simulink model "helicopter_auto_mode"  (Simulink 7.5)
settings: Solver=ode1  StartTime=0.0  StopTime=inf  FixedStep=0.1  RelTol=1e-3
PreLoadFcn:
  | load(fullfile(fileparts(which(bdroot)), 'object_types.mat'));
InitFcn:
  | load(fullfile(fileparts(which(bdroot)), 'object_types.mat'));
undefined symbols (not defined in the file or in its folder): HIL
libraries: quarc_library x4, simulink x1
settings Model: Creator=ovidiua  LastModifiedBy=ovidiua  SimulationMode=external  ExtModeTrigDuration=5000
settings SolverCC: PositivePriorityOrder=on
settings RTWCC: SystemTargetFile=quarc_windows.tlc  TemplateMakefile=quarc_default_tmf  Description=QUARC Win32 Target  ProcessScript=quarc_windows_make_rtw_hook
settings STFCustomTargetCC: TargetPreCompLibLocation=C:\PROGRA~2\QUARC\lib\2010a\windows\release  GeneratePreprocessorConditionals=Disable all  SystemTargetFile=quarc_windows.tlc
settings GRTTargetCC: TargetPreCompLibLocation=C:\PROGRA~2\QUARC\lib\2010a\windows\release  ParMdlRefBuildCompliant=off  CompOptLevelCompliant=off  MatFileLogging=off  ExtMode=on  ExtModeMexFile=quarc_comm

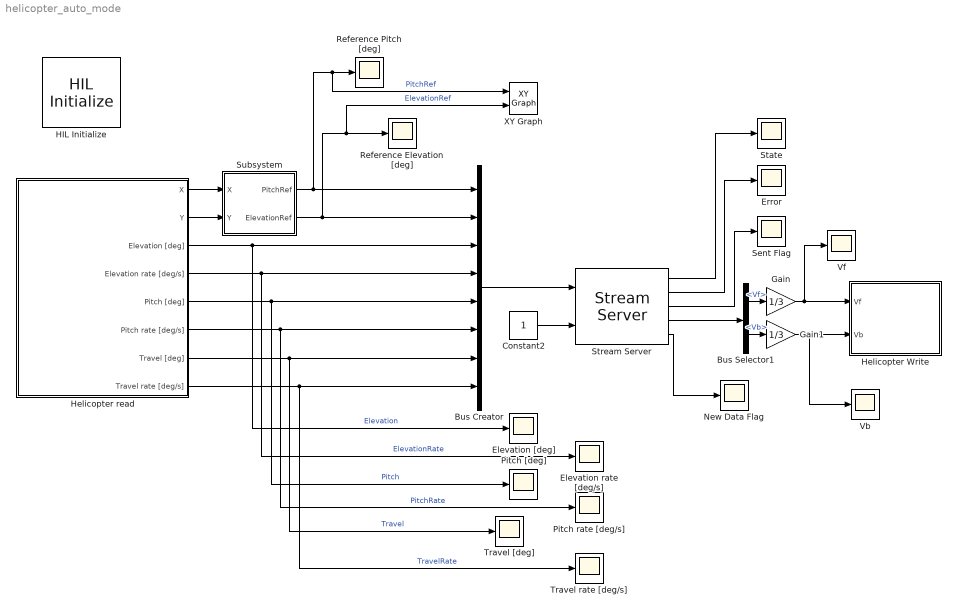
== system helicopter_auto_mode ==
  Bus Creator : BusCreator  Inputs='PitchRef','ElevationRef','Elevation','ElevationRate','Pitch','PitchRate','Travel','TravelRate'  UseBusObject=on
      settings: BusObject=BusObjectStates
  Bus Selector1 : BusSelector  OutputSignals=Vf,Vb
  Constant2 : Constant  OutDataType=sfix(16)  OutScaling=2^0
  Elevation [deg] : Scope
      settings: TimeRange=60  YMin=-30  YMax=30  SaveName=ScopeData2
  Elevation rate [deg/s] : Scope
      settings: TimeRange=60  YMin=-100  YMax=100  SaveName=ScopeData5
  Error : Scope
      settings: YMin=-1  YMax=1  SaveName=ScopeData8
  Gain : Gain  Gain=1/3  ParameterDataType=fixdt(1, 16)  ParameterScaling=2^0  OutDataType=fixdt(1, 16)  OutScaling=2^0
  Gain1 : Gain  Gain=1/3  ParameterDataType=fixdt(1, 16)  ParameterScaling=2^0  OutDataType=fixdt(1, 16)  OutScaling=2^0
  HIL Initialize : quarc_library/Data Acquisition/Generic/Configuration/HIL Initialize  object_name=HIL-1  board_type=q4  board_number=0  exclusive=off  active=off  hardware_clocks=[0:1]  clock_modes=[0 0]  set_clock_params_at_start=on  set_clock_params_at_switch_in=off  analog_input_channels=[0:3]  analog_input_maximums=10  analog_input_minimums=-10  set_analog_input_params_at_start=off  set_analog_input_params_at_switch_in=off  analog_output_channels=[0:3]  analog_output_maximums=[10]  analog_output_minimums=[-10]  initial_analog_outputs=[0]  final_analog_outputs=[0]  watchdog_analog_outputs=0  set_analog_output_params_at_start=on  set_analog_output_params_at_switch_in=off  set_analog_outputs_at_start=on  set_analog_outputs_at_switch_in=off  set_analog_outputs_at_terminate=on  set_analog_outputs_at_switch_out=off  set_analog_outputs_on_watchdog=off  digital_input_channels=[]  digital_output_channels=[]  digital_output_configuration=[]  initial_digital_outputs=[1]  final_digital_outputs=[1]  watchdog_digital_outputs=[2]  set_digital_output_params_at_start=off  set_digital_output_params_at_switch_in=off  set_digital_outputs_at_start=on  set_digital_outputs_at_switch_in=off  set_digital_outputs_at_terminate=on  set_digital_outputs_at_switch_out=off  set_digital_outputs_on_watchdog=off  encoder_channels=[0:3]  quadrature=[4]  encoder_filter_frequency=(1/60e-9)/1  initial_encoder_counts=[0]  set_encoder_params_at_start=on  set_encoder_params_at_switch_in=off  set_encoder_counts_at_start=on  set_encoder_counts_at_switch_in=off  pwm_channels=[]  pwm_modes=[0]  pwm_frequency=(1/60e-9)/1024  pwm_configuration=[]  pwm_alignment=[]  pwm_polarity=[]  pwm_leading_deadband=[]  pwm_trailing_deadband=[]  initial_pwm_outputs=[0]  final_pwm_outputs=[0]  watchdog_pwm_outputs=[]  set_pwm_params_at_start=on  set_pwm_params_at_switch_in=off  set_pwm_outputs_at_start=on  set_pwm_outputs_at_switch_in=off  set_pwm_outputs_at_terminate=on  set_pwm_outputs_at_switch_out=off  set_pwm_outputs_on_watchdog=off  other_output_channels=[]  initial_other_outputs=[]  final_other_outputs=[]  watchdog_other_outputs=[]  set_other_outputs_at_start=off  set_other_outputs_at_switch_in=off  set_other_outputs_at_terminate=off  set_other_outputs_at_switch_out=off  set_other_outputs_on_watchdog=off
  Helicopter Write : Subsystem
  Helicopter read : Subsystem
  New Data Flag : Scope
      settings: YMin=-1  YMax=1  SaveName=ScopeData9
  Pitch [deg] : Scope
      settings: TimeRange=60  YMin=-60  YMax=60  SaveName=ScopeData3
  Pitch rate [deg/s] : Scope
      settings: TimeRange=60  YMin=-100  YMax=100  SaveName=ScopeData6
  Reference Elevation [deg] : Scope
      settings: YMin=-3.75  YMax=-0.5
  Reference Pitch [deg] : Scope
      settings: YMin=-27.5  YMax=0
  Sent Flag : Scope
      settings: SaveName=ScopeData12
  State : Scope
      settings: YMin=-1  YMax=1  SaveName=ScopeData13
  Stream Server : quarc_library/Communications/Basic/Stream Server  uri_source=Specify via dialog (do not evaluate)  uri=shmem://foobar:1  apply_uri_to_all_configs=on  send_buffer_size=1460  receive_buffer_size=1460  byte_order=little endian (Intel - LSB first)  optimization=Minimum latency  implementation=Use blocking I/O in a separate thread  send_options=Send most recent data  receive_options=Receive most recent data  send_fifo_size=1000  receive_fifo_size=1000  send_priority=0  receive_priority=0  default_value=default_inputs  sample_time=qc_get_step_size  active=on  data_type=Specify via dialog  type_expr=BusObjectIn
      settings: AttributesFormatString="\"shmem://foobar:1\""
  Subsystem : Subsystem
  Travel [deg] : Scope
      settings: TimeRange=60  YMin=-360  YMax=360  SaveName=ScopeData4
  Travel rate [deg/s] : Scope
      settings: TimeRange=60  YMin=-100  YMax=100  SaveName=ScopeData7
  Vb : Scope
      settings: YMin=-22.5  YMax=20  SaveName=ScopeData11
  Vf : Scope
      settings: YMin=-80  YMax=70  SaveName=ScopeData10
  XY Graph : simulink/Sinks/XY Graph  SystemSampleTime=-1  xmin=-60  xmax=60  ymin=-30  ymax=30  st=-1
  wires:
  Subsystem/1(PitchRef) -> Bus Creator/1, Reference Pitch [deg]/1, XY Graph/1  "PitchRef"
  Subsystem/2(ElevationRef) -> Bus Creator/2, Reference Elevation [deg]/1, XY Graph/2  "ElevationRef"
  Helicopter read/3(Elevation [deg]) -> Elevation [deg]/1, Bus Creator/3  "Elevation"
  Helicopter read/4(Elevation rate [deg/s]) -> Elevation rate [deg/s]/1, Bus Creator/4  "ElevationRate"
  Helicopter read/5(Pitch [deg]) -> Pitch [deg]/1, Bus Creator/5  "Pitch"
  Helicopter read/6(Pitch rate [deg/s]) -> Pitch rate [deg/s]/1, Bus Creator/6  "PitchRate"
  Helicopter read/7(Travel [deg]) -> Travel [deg]/1, Bus Creator/7  "Travel"
  Helicopter read/8(Travel rate [deg/s]) -> Travel rate [deg/s]/1, Bus Creator/8  "TravelRate"
  Stream Server/1 -> State/1
  Stream Server/2 -> Error/1
  Constant2/1 -> Stream Server/2
  Bus Creator/1 -> Stream Server/1
  Stream Server/3 -> Sent Flag/1
  Stream Server/5 -> New Data Flag/1
  Stream Server/4 -> Bus Selector1/1
  Bus Selector1/1 -> Gain/1  "<Vf>"
  Bus Selector1/2 -> Gain1/1  "<Vb>"
  Helicopter read/1(X) -> Subsystem/1(X)
  Helicopter read/2(Y) -> Subsystem/2(Y)
  Gain/1 -> Vf/1, Helicopter Write/1("Vf ")
  Gain1/1 -> Vb/1, Helicopter Write/2(Vb)

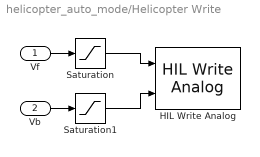
== system helicopter_auto_mode/Helicopter Write ==
  "Vf " : Inport
  Vb : Inport  Port=2
  HIL Write Analog : quarc_library/Data Acquisition/Generic/Immediate I//O/HIL Write Analog  object_name=HIL-1  channels=[0,1]  sample_time=-1  active=off  vector_input=off
  Saturation : Saturate  UpperLimit=3  LowerLimit=-3  OutDataType=fixdt(1, 16)  OutScaling=2^0
  Saturation1 : Saturate  UpperLimit=3  LowerLimit=-3  OutDataType=fixdt(1, 16)  OutScaling=2^0
  wires:
  Saturation/1 -> HIL Write Analog/1
  Saturation1/1 -> HIL Write Analog/2
  "Vf "/1 -> Saturation/1
  Vb/1 -> Saturation1/1

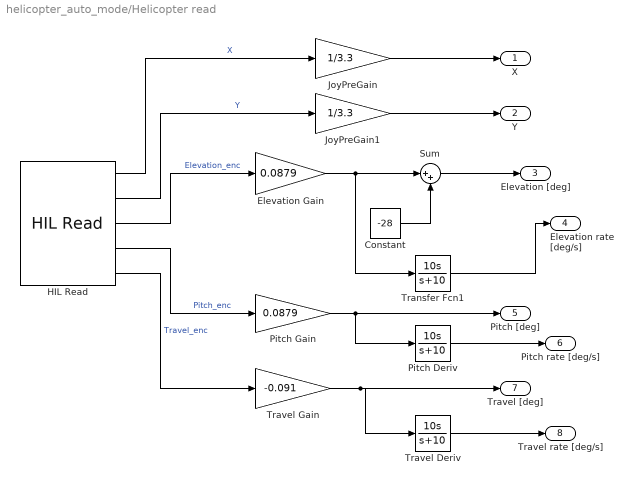
== system helicopter_auto_mode/Helicopter read ==
  Constant : Constant  Value=-28  OutDataType=fixdt(1, 16)  OutScaling=2^0
  Elevation Gain : Gain  Gain=0.0879  ParameterDataType=fixdt(1, 16)  ParameterScaling=2^0  OutDataType=fixdt(1, 16)  OutScaling=2^0
  HIL Read : quarc_library/Data Acquisition/Generic/Immediate I//O/HIL Read  object_name=HIL-1  analog_channels=[1:2]  encoder_channels=[2 1 0]  digital_channels=[]  other_channels=[]  sample_time=qc_get_step_size  active=on  vector_output=off  data_type_mode=Inherit via back propagation  encoder_data_type=double  digital_data_type=boolean
  JoyPreGain : Gain  Gain=1/3.3  ParameterDataType=fixdt(1, 16)  ParameterScaling=2^0  OutDataType=fixdt(1, 16)  OutScaling=2^0
  JoyPreGain1 : Gain  Gain=1/3.3  ParameterDataType=fixdt(1, 16)  ParameterScaling=2^0  OutDataType=fixdt(1, 16)  OutScaling=2^0
  Pitch Deriv : TransferFcn  Numerator=[10 0]  Denominator=[1 10]
  Pitch Gain : Gain  Gain=0.0879  ParameterDataType=fixdt(1, 16)  ParameterScaling=2^0  OutDataType=fixdt(1, 16)  OutScaling=2^0
  Sum : Sum  Inputs=|++  OutDataType=fixdt(1, 16)  OutScaling=2^0
  Transfer Fcn1 : TransferFcn  Numerator=[10 0]  Denominator=[1 10]
  Travel Deriv : TransferFcn  Numerator=[10 0]  Denominator=[1 10]
  Travel Gain : Gain  Gain=-0.091  ParameterDataType=fixdt(1, 16)  ParameterScaling=2^0  OutDataType=fixdt(1, 16)  OutScaling=2^0
  X : Outport
  Y : Outport  Port=2
  Elevation [deg] : Outport  Port=3
  Elevation rate [deg/s] : Outport  Port=4
  Pitch [deg] : Outport  Port=5
  Pitch rate [deg/s] : Outport  Port=6
  Travel [deg] : Outport  Port=7
  Travel rate [deg/s] : Outport  Port=8
  wires:
  Travel Gain/1 -> Travel Deriv/1, Travel [deg]/1
  Elevation Gain/1 -> Transfer Fcn1/1, Sum/1
  Pitch Gain/1 -> Pitch Deriv/1, Pitch [deg]/1
  Constant/1 -> Sum/2
  Travel Deriv/1 -> Travel rate [deg/s]/1
  Pitch Deriv/1 -> Pitch rate [deg/s]/1
  Sum/1 -> Elevation [deg]/1
  Transfer Fcn1/1 -> Elevation rate [deg/s]/1
  JoyPreGain1/1 -> Y/1
  JoyPreGain/1 -> X/1
  HIL Read/1 -> JoyPreGain/1  "X"
  HIL Read/2 -> JoyPreGain1/1  "Y"
  HIL Read/3 -> Elevation Gain/1  "Elevation_enc"
  HIL Read/4 -> Pitch Gain/1  "Pitch_enc"
  HIL Read/5 -> Travel Gain/1  "Travel_enc"

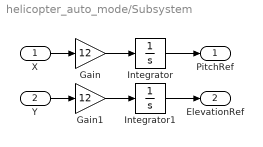
== system helicopter_auto_mode/Subsystem ==
  X : Inport
  Y : Inport  Port=2
  Gain : Gain  Gain=12  ParameterDataType=fixdt(1, 16)  ParameterScaling=2^0  OutDataType=fixdt(1, 16)  OutScaling=2^0
  Gain1 : Gain  Gain=12  ParameterDataType=fixdt(1, 16)  ParameterScaling=2^0  OutDataType=fixdt(1, 16)  OutScaling=2^0
  Integrator : Integrator  LimitOutput=on  UpperSaturationLimit=30  LowerSaturationLimit=-30  ContinuousStateAttributes='PitchReference'
  Integrator1 : Integrator  LimitOutput=on  UpperSaturationLimit=25  LowerSaturationLimit=-25  ContinuousStateAttributes='ElevationReference'
  PitchRef : Outport
  ElevationRef : Outport  Port=2
  wires:
  Gain/1 -> Integrator/1
  Gain1/1 -> Integrator1/1
  Integrator/1 -> PitchRef/1
  X/1 -> Gain/1
  Integrator1/1 -> ElevationRef/1
  Y/1 -> Gain1/1
